simulink model "PFMPC_dynamics_Compact"  (R2016a)
settings: Solver=ode4  StartTime=0.0  StopTime=300  FixedStep=Ts  RelTol=1e-3
values from neighbouring files (symbols this model uses):
  Ts = 0.1    [CPFMPC_Lyapunovbased.mat]    (also in CPFMPC_NoTerminalConstraint.mat; Coordination.m; Data_StrategyII_No_Constraint.mat; Data_StrategyI_Constraint.mat = 0.2)
libraries: simulink x1
settings Model: Creator=hung  LastModifiedBy=hung

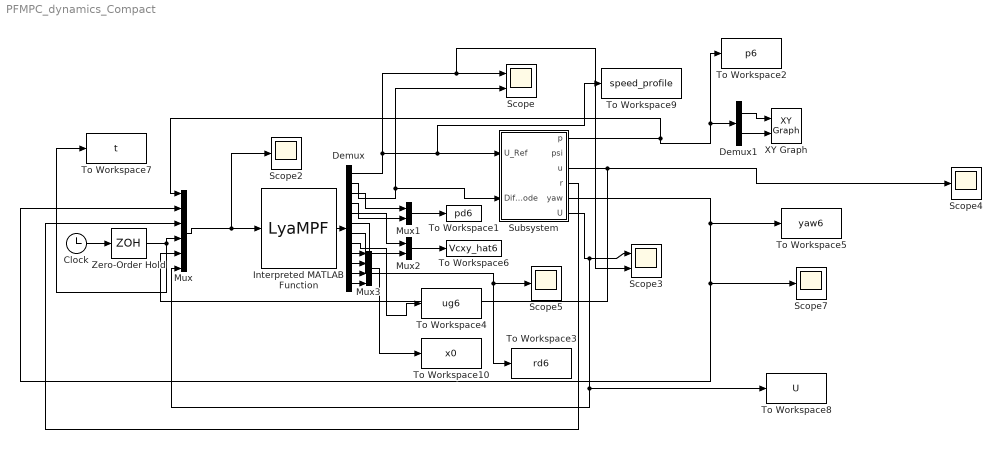
== system PFMPC_dynamics_Compact ==
  Clock : Clock
  Demux : Demux  Outputs=12
  Demux1 : Demux  Outputs=2
  Interpreted MATLAB Function : MATLABFcn  MATLABFcn=LyaMPF  OutputDimensions=12
  Mux : Mux  Inputs=6
  Mux1 : Mux  Inputs=2
  Mux2 : Mux  Inputs=2
  Mux3 : Mux
  Scope : Scope  NumInputPorts=2
  Scope{2,4..5,7} (4 alike) : Scope
  Scope3 : Scope  NumInputPorts=2
  Subsystem : Subsystem
  To Workspace1 : ToWorkspace  VariableName=pd6  SampleTime=Ts
  To Workspace10 : ToWorkspace  VariableName=x0  SampleTime=Ts
  To Workspace2 : ToWorkspace  VariableName=p6  SampleTime=Ts
  To Workspace3 : ToWorkspace  VariableName=rd6  SampleTime=Ts
  To Workspace4 : ToWorkspace  VariableName=ug6  SampleTime=Ts
  To Workspace5 : ToWorkspace  VariableName=yaw6  SampleTime=Ts
  To Workspace6 : ToWorkspace  VariableName=Vcxy_hat6  SampleTime=Ts
  To Workspace7 : ToWorkspace  VariableName=t  SampleTime=Ts
  To Workspace8 : ToWorkspace  VariableName=U  SampleTime=Ts
  To Workspace9 : ToWorkspace  VariableName=speed_profile  SampleTime=Ts
  XY Graph : simulink/Sinks/XY Graph  xmin=-80  xmax=80  ymin=-80  ymax=80  st=-1
  Zero-Order Hold : ZeroOrderHold  SampleTime=Ts
  wires:
  Interpreted MATLAB Function/1 -> Demux/1
  Demux/1 -> Scope3/2, Scope/1, To Workspace9/1, Subsystem/1(U_Ref)
  Demux/2 -> Scope/2, Subsystem/2(Diff_Mode)
  Mux/1 -> Scope2/1, Interpreted MATLAB Function/1
  Subsystem/1(p) -> To Workspace2/1, Demux1/1, Mux/1
  Clock/1 -> Zero-Order Hold/1
  Demux1/1 -> XY Graph/1
  Demux1/2 -> XY Graph/2
  Subsystem/3(u) -> Mux/5, Scope4/1
  Subsystem/5(yaw) -> Mux/2, Scope7/1, To Workspace5/1
  Zero-Order Hold/1 -> Mux/4, To Workspace7/1
  Subsystem/4(r) -> Mux/3
  Mux1/1 -> To Workspace1/1
  Demux/3 -> Mux1/1
  Demux/4 -> Mux1/2
  Subsystem/6(U) -> To Workspace8/1, Mux/6, Scope3/1
  Demux/7 -> Scope5/1, To Workspace3/1
  Mux2/1 -> To Workspace6/1
  Demux/5 -> Mux2/1
  Demux/6 -> Mux2/2
  Demux/8 -> To Workspace4/1
  Demux/9 -> Mux3/1
  Demux/10 -> Mux3/2
  Demux/11 -> Mux3/3
  Demux/12 -> Mux3/4
  Mux3/1 -> To Workspace10/1

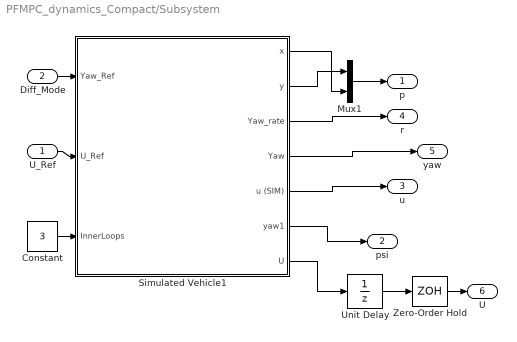
== system PFMPC_dynamics_Compact/Subsystem ==
  U_Ref : Inport
  Diff_Mode : Inport  Port=2
  Constant : Constant  Value=3
  Mux1 : Mux  Inputs=2
  Simulated Vehicle1 : Subsystem
  Unit Delay : UnitDelay  SampleTime=Ts
  Zero-Order Hold : ZeroOrderHold  SampleTime=Ts
  p : Outport
  psi : Outport  Port=2
  u : Outport  Port=3
  r : Outport  Port=4
  yaw : Outport  Port=5
  U : Outport  Port=6
  wires:
  Constant/1 -> Simulated Vehicle1/3(InnerLoops)
  U_Ref/1 -> Simulated Vehicle1/2(U_Ref)
  Diff_Mode/1 -> Simulated Vehicle1/1(Yaw_Ref)
  Mux1/1 -> p/1
  Simulated Vehicle1/2(y) -> Mux1/1
  Simulated Vehicle1/1(x) -> Mux1/2
  Simulated Vehicle1/3(Yaw_rate) -> r/1
  Simulated Vehicle1/4(Yaw) -> yaw/1
  Simulated Vehicle1/5(u (SIM)) -> u/1
  Simulated Vehicle1/6(yaw1) -> psi/1
  Unit Delay/1 -> Zero-Order Hold/1
  Zero-Order Hold/1 -> U/1
  Simulated Vehicle1/7(U) -> Unit Delay/1

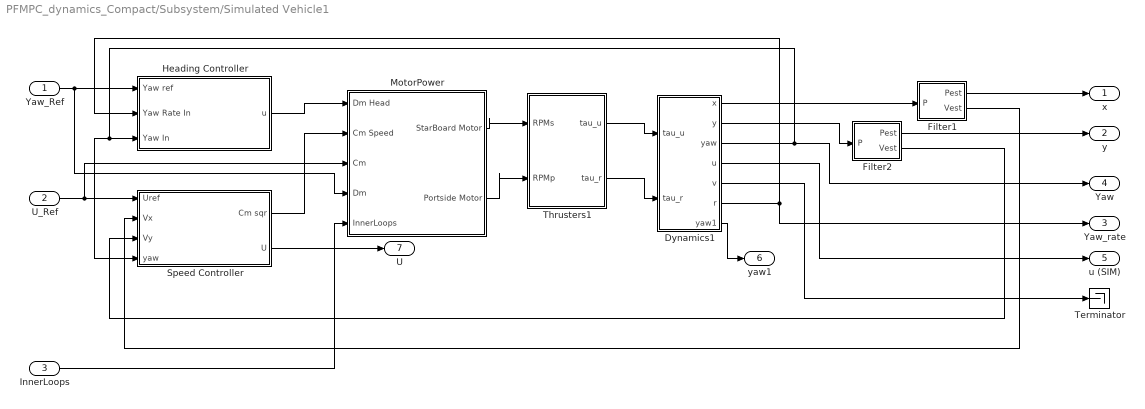
== system PFMPC_dynamics_Compact/Subsystem/Simulated Vehicle1 ==
  Yaw_Ref : Inport
  U_Ref : Inport  Port=2
  InnerLoops : Inport  Port=3
  Dynamics1 : Subsystem  mask{x0=5, y0=-10, yaw0=-pi/2, u0=0, v0=0, r0=0, dist_u=0, dist_v=0, dist_r=0, Vcx=0, Vcy=0}
      mask prompts: dist_u "Disturbance in u"; dist_v "Disturbance in v"; dist_r "Disturbance in r"; Vcx "Current x"; Vcy "Current y"
  Filter1 : Subsystem
  Filter2 : Subsystem
  Heading Controller : Subsystem  mask{Kp=45, Kd=110}
  MotorPower : Subsystem
  "Speed Controller " : Subsystem  mask{Kpu=60, Kiu=2, KSat=60}
      mask prompts: Kpu "Kp"; Kiu "Ki"; KSat "Common Mode Saturation"
  Terminator : Terminator
  Thrusters1 : Subsystem
  x : Outport
  y : Outport  Port=2
  Yaw_rate : Outport  Port=3
  Yaw : Outport  Port=4
  u (SIM) : Outport  Port=5
  yaw1 : Outport  Port=6
  U : Outport  Port=7
  wires:
  Thrusters1/1(tau_u) -> Dynamics1/1(tau_u)
  Thrusters1/2(tau_r) -> Dynamics1/2(tau_r)
  Dynamics1/1(x) -> Filter1/1(P)
  Dynamics1/2(y) -> Filter2/1(P)
  Dynamics1/3(yaw) -> Heading Controller/3(Yaw In), "Speed Controller "/4(yaw), Yaw/1
  MotorPower/1(StarBoard Motor) -> Thrusters1/1(RPMs)
  MotorPower/2(Portside Motor) -> Thrusters1/2(RPMp)
  Dynamics1/6(r) -> Heading Controller/2(Yaw Rate In), Yaw_rate/1
  Filter1/2(Vest) -> "Speed Controller "/2(Vx)
  Filter2/2(Vest) -> "Speed Controller "/3(Vy)
  "Speed Controller "/1(Cm sqr) -> MotorPower/2(Cm Speed)
  Yaw_Ref/1 -> Heading Controller/1(Yaw ref), MotorPower/4(Dm)
  Filter1/1(Pest) -> x/1
  Filter2/1(Pest) -> y/1
  U_Ref/1 -> "Speed Controller "/1(Uref), MotorPower/3(Cm)
  Heading Controller/1(u) -> MotorPower/1(Dm Head)
  InnerLoops/1 -> MotorPower/5(InnerLoops)
  Dynamics1/4(u) -> u (SIM)/1
  Dynamics1/5(v) -> Terminator/1
  Dynamics1/7(yaw1) -> yaw1/1
  "Speed Controller "/2(U) -> U/1

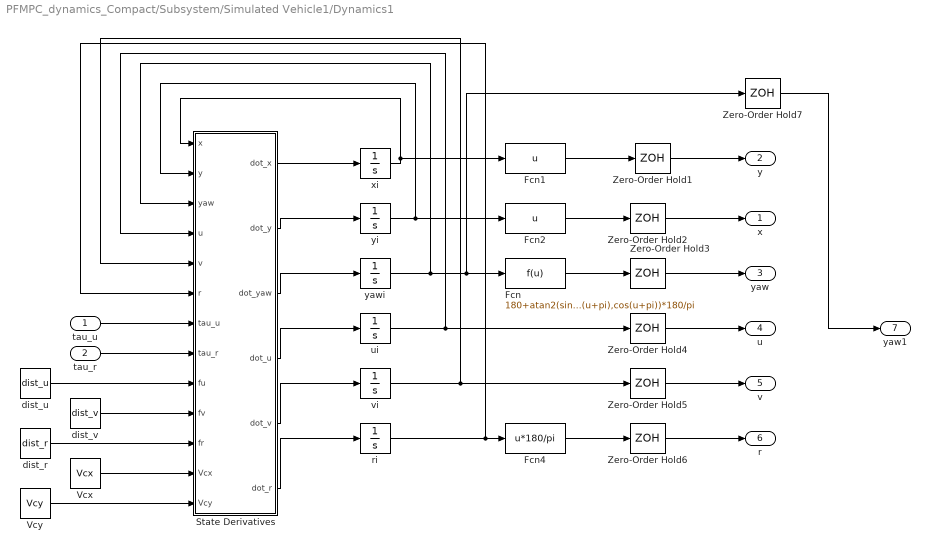
== system PFMPC_dynamics_Compact/Subsystem/Simulated Vehicle1/Dynamics1 ==
  tau_u : Inport
  tau_r : Inport  Port=2
  Fcn : Fcn  Expr=180+atan2(sin(u+pi),cos(u+pi))*180/pi
  Fcn1 : Fcn  Expr=u
  Fcn2 : Fcn  Expr=u
  Fcn4 : Fcn  Expr=u*180/pi
  State Derivatives : MATLAB Function  TreatAsAtomicUnit=on
  Vcx : Constant  Value=Vcx
  Vcy : Constant  Value=Vcy
  Zero-Order Hold{1..7} (7 alike) : ZeroOrderHold  SampleTime=Ts
  dist_r : Constant  Value=dist_r
  dist_u : Constant  Value=dist_u
  dist_v : Constant  Value=dist_v
  ri : Integrator  InitialCondition=r0
  ui : Integrator  InitialCondition=u0
  vi : Integrator  InitialCondition=v0
  xi : Integrator  InitialCondition=y0
  yawi : Integrator  InitialCondition=yaw0
  yi : Integrator  InitialCondition=x0
  x : Outport
  y : Outport  Port=2
  yaw : Outport  Port=3
  u : Outport  Port=4
  v : Outport  Port=5
  r : Outport  Port=6
  yaw1 : Outport  Port=7
  wires:
  Fcn4/1 -> Zero-Order Hold6/1
  State Derivatives/1(dot_x) -> xi/1
  State Derivatives/2(dot_y) -> yi/1
  State Derivatives/3(dot_yaw) -> yawi/1
  State Derivatives/4(dot_u) -> ui/1
  State Derivatives/5(dot_v) -> vi/1
  State Derivatives/6(dot_r) -> ri/1
  tau_u/1 -> State Derivatives/7(tau_u)
  yi/1 -> State Derivatives/2(y), Fcn2/1
  xi/1 -> State Derivatives/1(x), Fcn1/1
  ui/1 -> State Derivatives/4(u), Zero-Order Hold4/1
  ri/1 -> Fcn4/1, State Derivatives/6(r)
  vi/1 -> State Derivatives/5(v), Zero-Order Hold5/1
  tau_r/1 -> State Derivatives/8(tau_r)
  dist_u/1 -> State Derivatives/9(fu)
  dist_v/1 -> State Derivatives/10(fv)
  dist_r/1 -> State Derivatives/11(fr)
  yawi/1 -> Zero-Order Hold7/1, Fcn/1, State Derivatives/3(yaw)
  Vcx/1 -> State Derivatives/12(Vcx)
  Vcy/1 -> State Derivatives/13(Vcy)
  Fcn1/1 -> Zero-Order Hold1/1
  Fcn2/1 -> Zero-Order Hold2/1
  Zero-Order Hold1/1 -> y/1
  Zero-Order Hold2/1 -> x/1
  Zero-Order Hold3/1 -> yaw/1
  Zero-Order Hold4/1 -> u/1
  Zero-Order Hold5/1 -> v/1
  Zero-Order Hold6/1 -> r/1
  Fcn/1 -> Zero-Order Hold3/1
  Zero-Order Hold7/1 -> yaw1/1

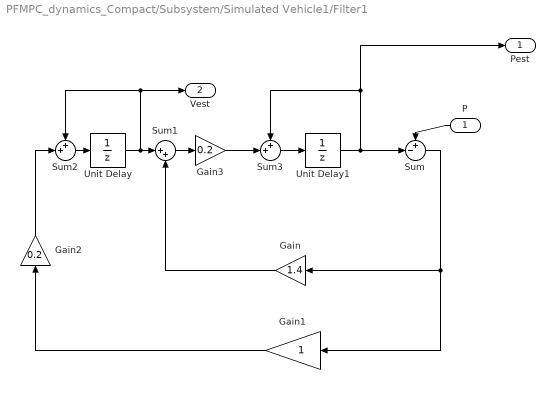
== system PFMPC_dynamics_Compact/Subsystem/Simulated Vehicle1/Filter1 ==
  P : Inport
  Gain : Gain  Gain=1.4
  Gain1 : Gain
  Gain2 : Gain  Gain=0.2
  Gain3 : Gain  Gain=0.2
  Sum : Sum  Inputs=+-|
  Sum1 : Sum  Inputs=|++
  Sum2 : Sum  Inputs=++|
  Sum3 : Sum  Inputs=++|
  Unit Delay : UnitDelay  SampleTime=Ts
  Unit Delay1 : UnitDelay  InitialCondition=5  SampleTime=Ts
  Pest : Outport
  Vest : Outport  Port=2
  wires:
  Sum3/1 -> Unit Delay1/1
  Unit Delay1/1 -> Pest/1, Sum3/1, Sum/2
  Gain3/1 -> Sum3/2
  Gain2/1 -> Sum2/2
  Sum2/1 -> Unit Delay/1
  P/1 -> Sum/1
  Gain1/1 -> Gain2/1
  Unit Delay/1 -> Vest/1, Sum2/1, Sum1/1
  Gain/1 -> Sum1/2
  Sum/1 -> Gain1/1, Gain/1
  Sum1/1 -> Gain3/1

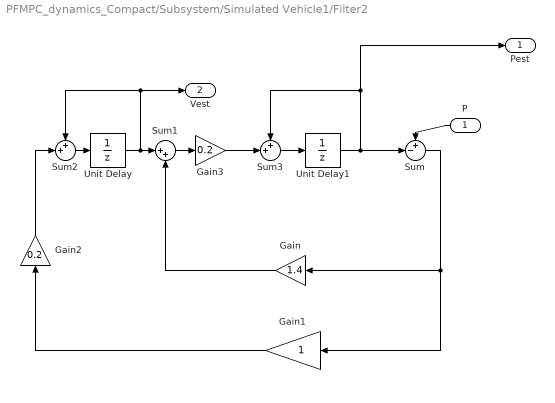
== system PFMPC_dynamics_Compact/Subsystem/Simulated Vehicle1/Filter2 ==
  P : Inport
  Gain : Gain  Gain=1.4
  Gain1 : Gain
  Gain2 : Gain  Gain=0.2
  Gain3 : Gain  Gain=0.2
  Sum : Sum  Inputs=+-|
  Sum1 : Sum  Inputs=|++
  Sum2 : Sum  Inputs=++|
  Sum3 : Sum  Inputs=++|
  Unit Delay : UnitDelay  SampleTime=Ts
  Unit Delay1 : UnitDelay  InitialCondition=-10  SampleTime=Ts
  Pest : Outport
  Vest : Outport  Port=2
  wires:
  Sum1/1 -> Gain3/1
  Sum/1 -> Gain/1, Gain1/1
  Gain/1 -> Sum1/2
  Unit Delay/1 -> Sum1/1, Sum2/1, Vest/1
  Gain1/1 -> Gain2/1
  P/1 -> Sum/1
  Sum2/1 -> Unit Delay/1
  Gain2/1 -> Sum2/2
  Gain3/1 -> Sum3/2
  Unit Delay1/1 -> Sum/2, Sum3/1, Pest/1
  Sum3/1 -> Unit Delay1/1

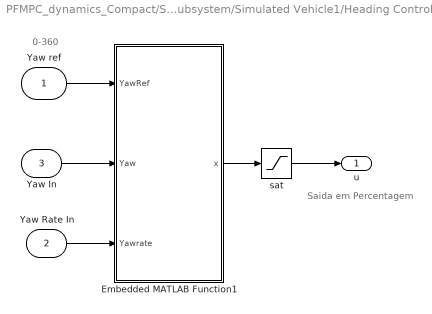
== system PFMPC_dynamics_Compact/Subsystem/Simulated Vehicle1/Heading Controller ==
  note: 0-360
  note: Saida em Percentagem
  Yaw ref : Inport  SampleTime=Ts
  Yaw Rate In : Inport  Port=2  SampleTime=Ts
  Yaw In : Inport  Port=3
  Embedded MATLAB Function1 : MATLAB Function  TreatAsAtomicUnit=on
  sat : Saturate  UpperLimit=Inf  LowerLimit=-Inf  SampleTime=Ts
  u : Outport
  wires:
  Yaw ref/1 -> Embedded MATLAB Function1/1(YawRef)
  Embedded MATLAB Function1/1(x) -> sat/1
  Yaw In/1 -> Embedded MATLAB Function1/2(Yaw)
  Yaw Rate In/1 -> Embedded MATLAB Function1/3(Yawrate)
  sat/1 -> u/1

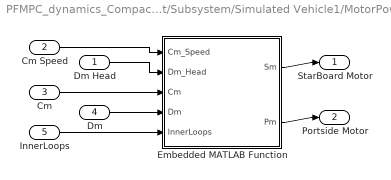
== system PFMPC_dynamics_Compact/Subsystem/Simulated Vehicle1/MotorPower ==
  Dm Head : Inport
  Cm Speed : Inport  Port=2
  Cm : Inport  Port=3
  Dm : Inport  Port=4
  InnerLoops : Inport  Port=5
  Embedded MATLAB Function : MATLAB Function  TreatAsAtomicUnit=on
  StarBoard Motor : Outport
  Portside Motor : Outport  Port=2
  wires:
  Embedded MATLAB Function/2(Pm) -> Portside Motor/1
  Embedded MATLAB Function/1(Sm) -> StarBoard Motor/1
  Dm Head/1 -> Embedded MATLAB Function/2(Dm_Head)
  Cm Speed/1 -> Embedded MATLAB Function/1(Cm_Speed)
  Cm/1 -> Embedded MATLAB Function/3(Cm)
  Dm/1 -> Embedded MATLAB Function/4(Dm)
  InnerLoops/1 -> Embedded MATLAB Function/5(InnerLoops)

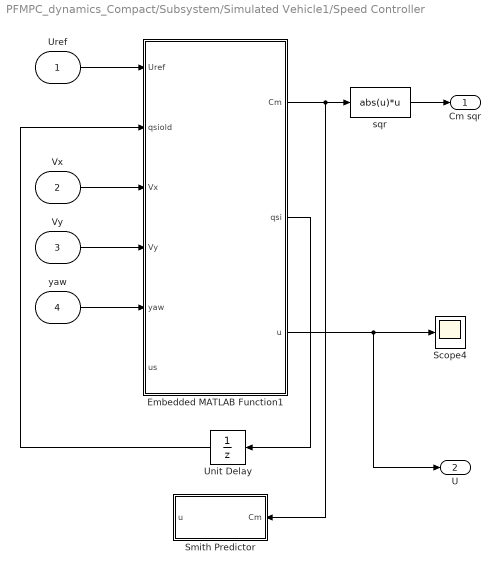
== system PFMPC_dynamics_Compact/Subsystem/Simulated Vehicle1/Speed Controller  ==
  Uref : Inport
  Vx : Inport  Port=2
  Vy : Inport  Port=3
  yaw : Inport  Port=4
  Embedded MATLAB Function1 : MATLAB Function  TreatAsAtomicUnit=on
  Scope4 : Scope
  Smith Predictor : Subsystem
  Unit Delay : UnitDelay  SampleTime=Ts
  sqr : Fcn  Expr=abs(u)*u
  Cm sqr : Outport
  U : Outport  Port=2
  wires:
  Embedded MATLAB Function1/3(u) -> U/1, Scope4/1
  yaw/1 -> Embedded MATLAB Function1/5(yaw)
  Vy/1 -> Embedded MATLAB Function1/4(Vy)
  Vx/1 -> Embedded MATLAB Function1/3(Vx)
  Embedded MATLAB Function1/1(Cm) -> Smith Predictor/1(Cm), sqr/1
  Uref/1 -> Embedded MATLAB Function1/1(Uref)
  Embedded MATLAB Function1/2(qsi) -> Unit Delay/1
  Unit Delay/1 -> Embedded MATLAB Function1/2(qsiold)
  sqr/1 -> Cm sqr/1

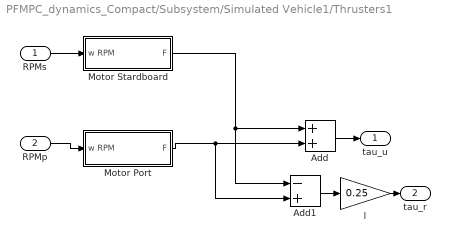
== system PFMPC_dynamics_Compact/Subsystem/Simulated Vehicle1/Thrusters1 ==
  RPMs : Inport
  RPMp : Inport  Port=2
  Add : Sum
  Add1 : Sum  Inputs=-+
  Motor Port : Subsystem  mask{K0=7.2115, tau=0.346, eta=4/(1500^2)}
      mask prompts: tau "Atraso do Motor"; eta "Constante de conversao W-F"
  Motor Stardboard : Subsystem  mask{K0=7.2115, tau=0.346, eta=4/(1500^2)}
      mask prompts: tau "Atraso do Motor"; eta "Constante de conversao W-F"
  l : Gain  Gain=0.25
  tau_u : Outport
  tau_r : Outport  Port=2
  wires:
  Add1/1 -> l/1
  RPMs/1 -> Motor Stardboard/1(w RPM)
  Add/1 -> tau_u/1
  RPMp/1 -> Motor Port/1(w RPM)
  l/1 -> tau_r/1
  Motor Port/1(F) -> Add/2, Add1/2
  Motor Stardboard/1(F) -> Add/1, Add1/1

== system PFMPC_dynamics_Compact/Subsystem/Simulated Vehicle1/Speed Controller /Smith Predictor ==
  Cm : Inport
  Common mode to u : DiscreteTransferFcn  Numerator=[0.0006641 0]  Denominator=[1 -0.6368 -0.2936]  SampleTime=Ts
  Integer Delay2 : Delay  DelayLength=7  InputProcessing=Inherited  SampleTime=Ts
  Sum2 : Sum  Inputs=|-+
  u : Outport
  wires:
  Cm/1 -> Common mode to u/1
  Common mode to u/1 -> Integer Delay2/1, Sum2/2
  Integer Delay2/1 -> Sum2/1
  Sum2/1 -> u/1

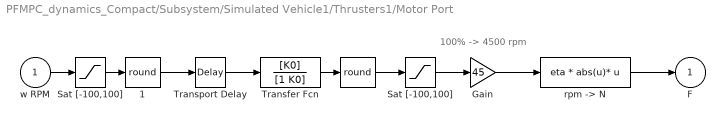
== system PFMPC_dynamics_Compact/Subsystem/Simulated Vehicle1/Thrusters1/Motor Port ==
  note: 100% -> 4500 rpm
  w RPM : Inport
  "  " : Rounding  Operator=round
  "  1" : Rounding  Operator=round
  Gain : Gain  Gain=45
  Sat [-100,100] : Saturate  UpperLimit=100  LowerLimit=-100
  "Sat [-100,100] " : Saturate  UpperLimit=100  LowerLimit=-100
  Transfer Fcn : TransferFcn  Numerator=[K0]  Denominator=[1 K0]
  Transport Delay : TransportDelay  DelayTime=tau
  "rpm -> N" : Fcn  Expr=eta * abs(u)* u
  F : Outport
  wires:
  Transfer Fcn/1 -> "  "/1
  Transport Delay/1 -> Transfer Fcn/1
  "  1"/1 -> Transport Delay/1
  "  "/1 -> "Sat [-100,100] "/1
  "rpm -> N"/1 -> F/1
  Sat [-100,100]/1 -> "  1"/1
  Gain/1 -> "rpm -> N"/1
  w RPM/1 -> Sat [-100,100]/1
  "Sat [-100,100] "/1 -> Gain/1

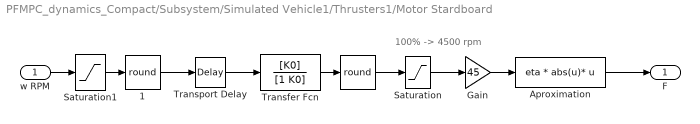
== system PFMPC_dynamics_Compact/Subsystem/Simulated Vehicle1/Thrusters1/Motor Stardboard ==
  note: 100% -> 4500 rpm
  w RPM : Inport
  "  " : Rounding  Operator=round
  "  1" : Rounding  Operator=round
  Aproximation : Fcn  Expr=eta * abs(u)* u
  Gain : Gain  Gain=45
  Saturation : Saturate  UpperLimit=100  LowerLimit=-100
  Saturation1 : Saturate  UpperLimit=100  LowerLimit=-100
  Transfer Fcn : TransferFcn  Numerator=[K0]  Denominator=[1 K0]
  Transport Delay : TransportDelay  DelayTime=tau
  F : Outport
  wires:
  Transfer Fcn/1 -> "  "/1
  Transport Delay/1 -> Transfer Fcn/1
  "  1"/1 -> Transport Delay/1
  "  "/1 -> Saturation/1
  Aproximation/1 -> F/1
  Saturation1/1 -> "  1"/1
  Gain/1 -> Aproximation/1
  w RPM/1 -> Saturation1/1
  Saturation/1 -> Gain/1

== matlab function PFMPC_dynamics_Compact/Subsystem/Simulated Vehicle1/Dynamics1/State Derivatives ==
  data: x input; y input; yaw input; u input; v input; r input; tau_u input; dot_x output; tau_r input; dot_y output; dot_yaw output; dot_u output; dot_v output; dot_r output; fu input; fv input; fr input; Vcx input; Vcy input
function [dot_x,dot_y,dot_yaw,dot_u,dot_v,dot_r] = fcn(x,y,yaw,u,v,r,tau_u,tau_r,fu,fv,fr, Vcx, Vcy)
%state = [x, y, yaw, u, v, r]

% %%%%%% Coefficients
% mass = 17.0;
% I_z = 4.14;
% X_dot_u = -20;
% Y_dot_v = -1.3175;
% N_dot_r =  -8.69;
% X_u = -0.2;
% Y_v = -55.117;
% N_r = -4.14;
% X_uu = -25; 
% Y_vv = -101.2776;
% N_rr = -6.23;

%%%%%% Coefficients
mass = 17.0;
I_z = 1;
X_dot_u = -20;
Y_dot_v = -30;%-1.3175;
N_dot_r = -8.69;% -0.5;
X_u = -0.2;
Y_v = -50;
N_r = -4.14; %-0.1
X_uu = -25; 
Y_vv = -0.01;%-101.2776;
N_rr = -6.23; %-21

%%%%%% masses
m_u = mass - X_dot_u;
m_v = mass - Y_dot_v;
m_r = I_z - N_dot_r;
m_uv = m_u - m_v;

%%%%%%%%% drag

d_u = -X_u - X_uu*abs(u);
d_v = -Y_v - Y_vv*abs(v);
d_r = -N_r - N_rr*abs(r);

%%%%%%%%% Dynamics

dot_u = 1/m_u*(tau_u + m_v*v*r - d_u*u+fu);
dot_v = 1/m_v*(-m_u*u*r - d_v*v+fv);
dot_r = 1/m_r*(tau_r + m_uv*u*v - d_r*r+fr);

dot_x = u*cos(yaw) - v*sin(yaw) + Vcx;
dot_y = u*sin(yaw) + v*cos(yaw) + Vcy;
dot_yaw = r;

== matlab function PFMPC_dynamics_Compact/Subsystem/Simulated Vehicle1/Heading Controller/Embedded MATLAB Function1 ==
  data: YawRef input; x output; Yaw input; Yawrate input; Kd parameter; Kp parameter
function x = controller(YawRef, Yaw, Yawrate, Kd, Kp)
err = ( YawRef- Yaw );
if(err>180) 
     err=err-360;
elseif(err<-180) 
     err=360+err;
end

x=Kp*err-Kd*Yawrate;

== matlab function PFMPC_dynamics_Compact/Subsystem/Simulated Vehicle1/MotorPower/Embedded MATLAB Function ==
  data: Sm output; Pm output; Cm_Speed input; Dm_Head input; Cm input; Dm input; InnerLoops input
function [Sm,Pm] = fcn(Cm_Speed, Dm_Head, Cm, Dm, InnerLoops)
Cm_sqr=0;
Dm_sqr=0;
switch InnerLoops
    case 0
        ; % Don't do anything
    case 1
        Cm_sqr=Cm_Speed;
        Dm_sqr=Dm_Head;
    case 2
        Cm_sqr=Cm*abs(Cm);
        Dm_sqr=Dm_Head;
    case 3
        Cm_sqr=Cm_Speed;
        Dm_sqr=Dm*abs(Dm);
    case 4
        Cm_sqr=Cm*abs(Cm);
        Dm_sqr=Dm*abs(Dm);
    otherwise
end

Pm = round(sqrt(abs(Cm_sqr+Dm_sqr))*sign(Cm_sqr+Dm_sqr));
Sm = round(sqrt(abs(Cm_sqr-Dm_sqr))*sign(Cm_sqr-Dm_sqr));

== matlab function PFMPC_dynamics_Compact/Subsystem/Simulated Vehicle1/Speed Controller /Embedded MATLAB Function1 ==
  data: Cm output; Uref input; Kpu parameter; Kiu parameter; qsiold input; qsi output; Vx input; Vy input; yaw input; u output; us input; KSat parameter
function [Cm, qsi, u] = controller(Uref, Kpu,Kiu, qsiold,Vx,Vy,yaw, us, KSat)
u=Vx*sind(yaw)+Vy*cosd(yaw);
err=u-Uref;
qsi=qsiold+err;

Cm=-Kpu*(err+us)-Kiu*qsi;
% Cm =+40*Uref-Kiu*qsi;
% if(t>10)
%     qsi=qsiold+err;
%     Cm =-Kpu*err-Kiu*qsi;
% end
if(abs(Cm) >= KSat)
   Cm = KSat*sign(Cm); 
   qsi = qsiold;
end
